simulink model "caravan"  (R2023a)
settings: Solver=VariableStepAuto  StartTime=0.0  StopTime=100  RelTol=1e-3
values from neighbouring files (symbols this model uses):
  aeroDragCoeff = 0.18    [run_model.m]
  airDensity = 1.293    [run_model.m]
  frontArea = 3    [run_model.m]
  gravity = 9.81    [run_model.m]
  inertialMassSPC = (massSPC + nTires * inertia_tire / radiusTire^2) * towing_ratio    (= 995.625)    [run_model.m]
  massSPC = massBatt + massCaravan + massStorage + nTires * massTire    (= 975.625)    [run_model.m]
  rollingResistCoeff = 0.008    [run_model.m]
undefined symbols (not defined in the file or in its folder): magnitude
libraries: simulink x1
settings Model: Creator=jonathan  LastModifiedBy=sandu
settings OptimizationCC: ReuseModelBlockBuffer=off

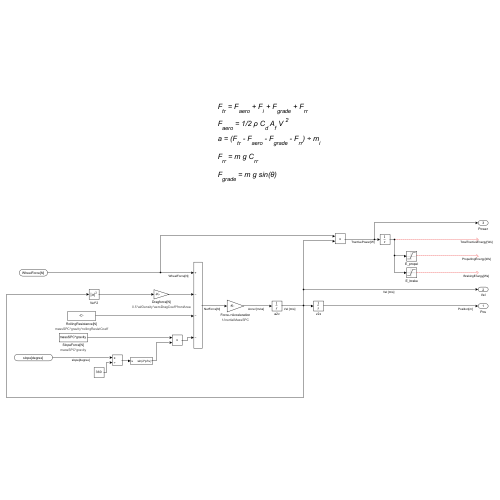
[thumbnail: Simulink's stored preview of the top-level diagram]
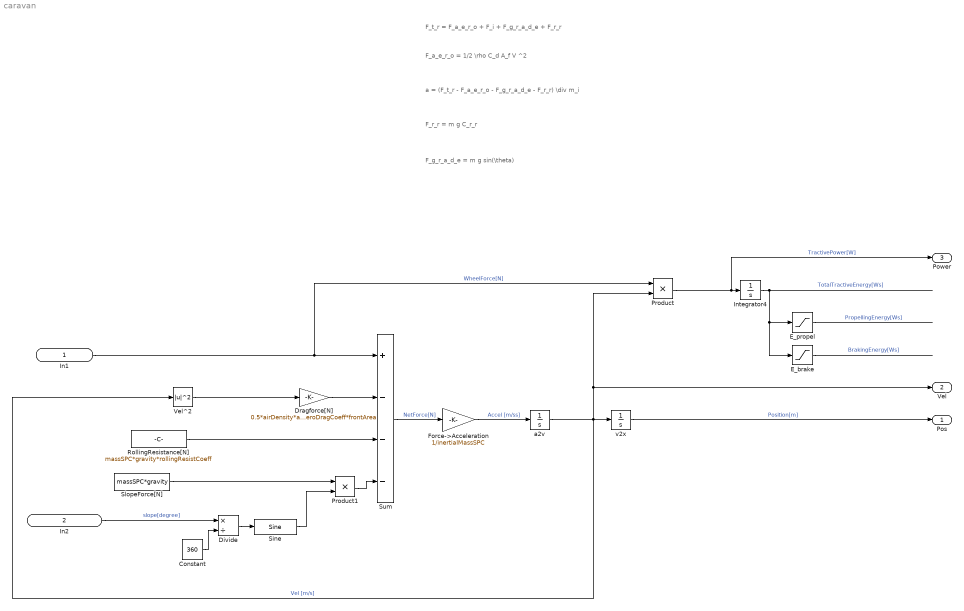
== system caravan ==
  note: F_g_r_a_d_e = m g sin(\theta)
  note: F_a_e_r_o = 1/2 \rho C_d A_f V ^2
  note: a = (F_t_r - F_a_e_r_o - F_g_r_a_d_e - F_r_r) \div m_i
  note: F_t_r = F_a_e_r_o + F_i + F_g_r_a_d_e + F_r_r
  note: F_r_r = m g C_r_r
  In1 : Inport  Unit=N
  In2 : Inport  Port=2
  Constant : Constant  Value=360
  Divide : Product  Inputs=*/
  Dragforce[N] : Gain  Gain=0.5*airDensity*aeroDragCoeff*frontArea
      settings: AttributesFormatString=%<Gain>
  E_brake : Saturate  UpperLimit=0  LowerLimit=-inf
  E_propel : Saturate  UpperLimit=inf  LowerLimit=0
  Force->Acceleration : Gain  Gain=1/inertialMassSPC
      settings: AttributesFormatString=%<Gain>
  Integrator4 : Integrator
  Product : Product
  Product1 : Product
  RollingResistance[N] : Constant  Value=massSPC*gravity*rollingResistCoeff
      settings: AttributesFormatString=%<Value>
  Sine : simulink/Lookup Tables/Sine  Formula=sin(2*pi*u)  NumDataPoints=(2^5)+1  OutputWordLength=16  InternalRulePriority=Speed
  SlopeForce[N] : Constant  Value=massSPC*gravity
      settings: AttributesFormatString=%<Value>
  Sum : Sum  Inputs=+---
  Vel^2 : Math  Operator=magnitude^2  SignedPower=on
  a2v : Integrator
  v2x : Integrator
  Pos : Outport
  Vel : Outport  Port=2
  Power : Outport  Port=3
  wires:
  Vel^2/1 -> Dragforce[N]/1
  Sum/1 -> Force->Acceleration/1  "NetForce[N]"
  v2x/1 -> Pos/1  "Position[m]"
  Dragforce[N]/1 -> Sum/2
  Integrator4/1 -> E_propel/1, E_brake/1  "TotalTractiveEnergy[Ws]"
  E_propel/1 -> ?  "PropellingEnergy[Ws]"
  a2v/1 -> Vel/1, Product/2, Vel^2/1, v2x/1  "Vel [m/s]"
  In1/1 -> Product/1, Sum/1  "WheelForce[N]"
  Product/1 -> Power/1, Integrator4/1  "TractivePower[W]"
  E_brake/1 -> ?  "BrakingEnergy[Ws]"
  Force->Acceleration/1 -> a2v/1  "Accel [m/ss]"
  RollingResistance[N]/1 -> Sum/3
  Product1/1 -> Sum/4
  SlopeForce[N]/1 -> Product1/1
  Sine/1 -> Product1/2
  Divide/1 -> Sine/1
  In2/1 -> Divide/1  "slope[degree]"
  Constant/1 -> Divide/2
